simulink model "softarm_flying_contact_demo"  (R2025a)
settings: Solver=ode15s  StartTime=0.0  StopTime=1  RelTol=1e-3
PreLoadFcn:
  | softarm_root=fileparts(get_param(bdroot,'FileName'));addpath(softarm_root);addpath(fullfile(softarm_root,'matlab'));
InitFcn:
  | softarm_root=fileparts(get_param(bdroot,'FileName'));addpath(fullfile(softarm_root,'matlab'));softarm.initModel(fullfile(softarm_root,'examples','generated','pcc_flying_plane_contact_n1'));
undefined symbols (not defined in the file or in its folder): softarm_narm, softarm_nc
settings Model: Creator=rlwan  LastModifiedBy=rlwan

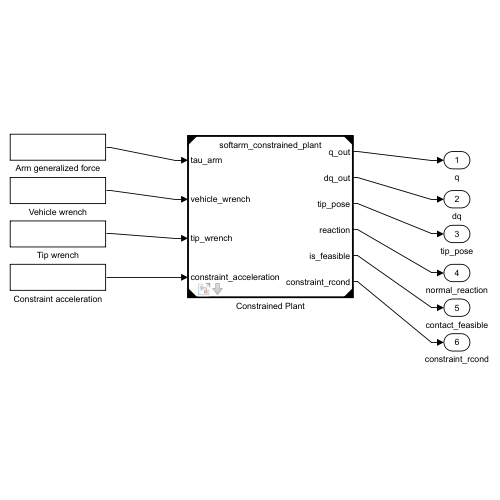
[thumbnail: Simulink's stored preview of the top-level diagram]
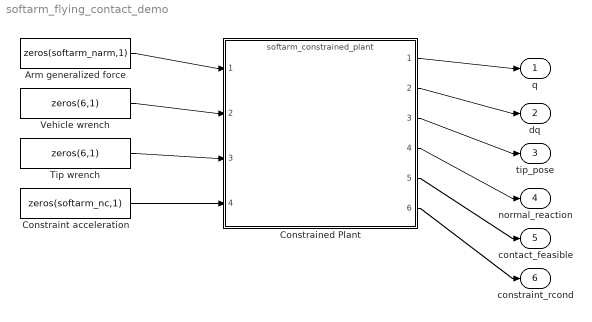
== system softarm_flying_contact_demo ==
  Arm generalized force : Constant  Value=zeros(softarm_narm,1)
  Constrained Plant : ModelReference  ModelNameDialog=softarm_constrained_plant  ParameterArgumentNames=Bundle  ParameterArgumentValues=Bundle  UsingDefaultArgumentValue=0  ModelReferenceVersion=1.1  Bundle='examples/generated/pcc_flying_plane_contact_n1'
  Constraint acceleration : Constant  Value=zeros(softarm_nc,1)
  Tip wrench : Constant  Value=zeros(6,1)
  Vehicle wrench : Constant  Value=zeros(6,1)
  q : Outport
  dq : Outport  Port=2
  tip_pose : Outport  Port=3
  normal_reaction : Outport  Port=4
  contact_feasible : Outport  Port=5
  constraint_rcond : Outport  Port=6
  wires:
  Constrained Plant/1 -> q/1
  Constrained Plant/2 -> dq/1
  Constrained Plant/3 -> tip_pose/1
  Constrained Plant/4 -> normal_reaction/1
  Constrained Plant/5 -> contact_feasible/1
  Constrained Plant/6 -> constraint_rcond/1
  Arm generalized force/1 -> Constrained Plant/1
  Vehicle wrench/1 -> Constrained Plant/2
  Tip wrench/1 -> Constrained Plant/3
  Constraint acceleration/1 -> Constrained Plant/4
